simulink model "Ellipse"  (R2023a)
settings: Solver=FixedStepAuto  StartTime=0.0  StopTime=20  FixedStep=0.005  RelTol=1e-3
values from neighbouring files (symbols this model uses):
  step_height = 0.06    [InitialisationScript.m]    (also in simulation_setup.m)
  step_length = 0.04    [InitialisationScript.m]    (also in simulation_setup.m)
libraries: simulink_extras x2
settings Model: Creator=basti  LastModifiedBy=basti
settings SolverCC: EnableFixedStepZeroCrossing=on

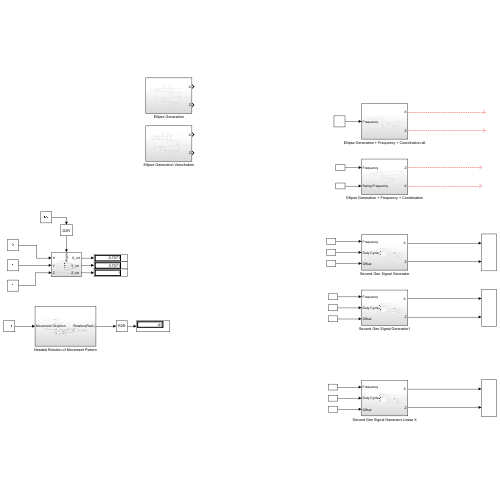
[thumbnail: Simulink's stored preview of the top-level diagram]
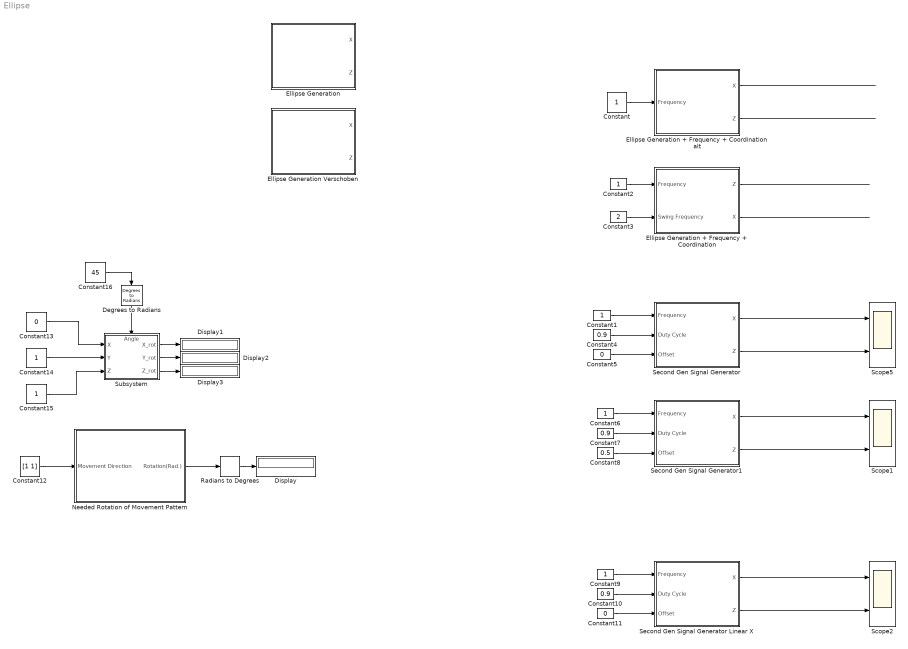
== system Ellipse ==
  Constant{,1..2,6,9,14..15} (7 alike) : Constant
  Constant10 : Constant  Value=0.9
  Constant11 : Constant  Value=0
  Constant12 : Constant  Value=[1 1]
  Constant13 : Constant  Value=0
  Constant16 : Constant  Value=45
  Constant3 : Constant  Value=2
  Constant4 : Constant  Value=0.9
  Constant5 : Constant  Value=0
  Constant7 : Constant  Value=0.9
  Constant8 : Constant  Value=0.5
  Degrees to Radians : simulink_extras/Transformations/Degrees to Radians
  Display{,1..3} (4 alike) : Display
  Ellipse Generation : Subsystem
  Ellipse Generation + Frequency + Coordination : Subsystem
  Ellipse Generation + Frequency + Coordination alt : Subsystem
  Ellipse Generation Verschoben : Subsystem
  Needed Rotation of Movement Pattern : Subsystem
  Radians to Degrees : simulink_extras/Transformations/Radians to Degrees
  Scope1 : Scope  NumInputPorts=2
  Scope2 : Scope  NumInputPorts=2
  Scope5 : Scope  NumInputPorts=2
  Second Gen Signal Generator : Subsystem
  Second Gen Signal Generator Linear X : Subsystem
  Second Gen Signal Generator1 : Subsystem
  Subsystem : Subsystem
      settings: PortSchema="{\"entries\":[{\"content\":{\"sides\":[{\"content\":{\"connectorIds\":[\"In1\",\"In2\",\"In3\"]},\"type\":\"ConnectorPlacement.EquallySpacedRectSide\",\"uuid\":\"84b9b2e7-3aec-4c44-82b0-943baf46ecad\"},{\"content\":{\"connectorIds\":[\"Out1\",\"Out2\",\"Out3\"],\"side\":\"RIGHT\"},\"type\":\"ConnectorPlacement.EquallySpacedRectSide\",\"uuid\":\"b6460351-c898-40bb-b6f7-4663874c85b4\"},{\"content\":{\"connectorIds\":[\"In4\"],\"side\":\"TOP\"},\"type\":\"ConnectorPlacement.EquallySpacedRectSide\",\"uuid\":\"52dfc046-6500-4cf8-9639-535088e7a0e1\"}]},\"type\":\"ConnectorPlacement.EquallySpacedConnector\",\"uuid\":\"f9a3b501-bdbb-45c4-9129-59c2d41cd802\"}],\"packageUris\":[\"http://schema.mathworks.com/mf0/Connector/R2020b\"],\"version\":\"1.0\"}"
  wires:
  Ellipse Generation + Frequency + Coordination alt/1(X) -> ?
  Ellipse Generation + Frequency + Coordination alt/2(Z) -> ?
  Constant/1 -> Ellipse Generation + Frequency + Coordination alt/1(Frequency)
  Constant3/1 -> Ellipse Generation + Frequency + Coordination/2(Swing Frequency)
  Constant2/1 -> Ellipse Generation + Frequency + Coordination/1(Frequency)
  Ellipse Generation + Frequency + Coordination/1(Z) -> ?
  Ellipse Generation + Frequency + Coordination/2(X) -> ?
  Constant1/1 -> Second Gen Signal Generator/1(Frequency)
  Constant4/1 -> Second Gen Signal Generator/2(Duty Cycle)
  Constant5/1 -> Second Gen Signal Generator/3(Offset)
  Second Gen Signal Generator/1("X ") -> Scope5/1
  Second Gen Signal Generator/2(Z) -> Scope5/2
  Constant6/1 -> Second Gen Signal Generator1/1(Frequency)
  Constant8/1 -> Second Gen Signal Generator1/3(Offset)
  Constant7/1 -> Second Gen Signal Generator1/2(Duty Cycle)
  Second Gen Signal Generator1/1("X ") -> Scope1/1
  Second Gen Signal Generator1/2(Z) -> Scope1/2
  Constant11/1 -> Second Gen Signal Generator Linear X/3(Offset)
  Constant10/1 -> Second Gen Signal Generator Linear X/2(Duty Cycle)
  Constant9/1 -> Second Gen Signal Generator Linear X/1(Frequency)
  Second Gen Signal Generator Linear X/2(Z) -> Scope2/2
  Second Gen Signal Generator Linear X/1("X ") -> Scope2/1
  Needed Rotation of Movement Pattern/1(Rotation(Rad.)) -> Radians to Degrees/1
  Radians to Degrees/1 -> Display/1
  Constant12/1 -> Needed Rotation of Movement Pattern/1(Movement Direction)
  Constant13/1 -> Subsystem/1("X ")
  Constant14/1 -> Subsystem/2(Y)
  Constant15/1 -> Subsystem/3(Z)
  Subsystem/1(X_rot) -> Display1/1
  Subsystem/2("Y_rot ") -> Display2/1
  Subsystem/3("Z_rot ") -> Display3/1
  Constant16/1 -> Degrees to Radians/1
  Degrees to Radians/1 -> Subsystem/4(Angle)

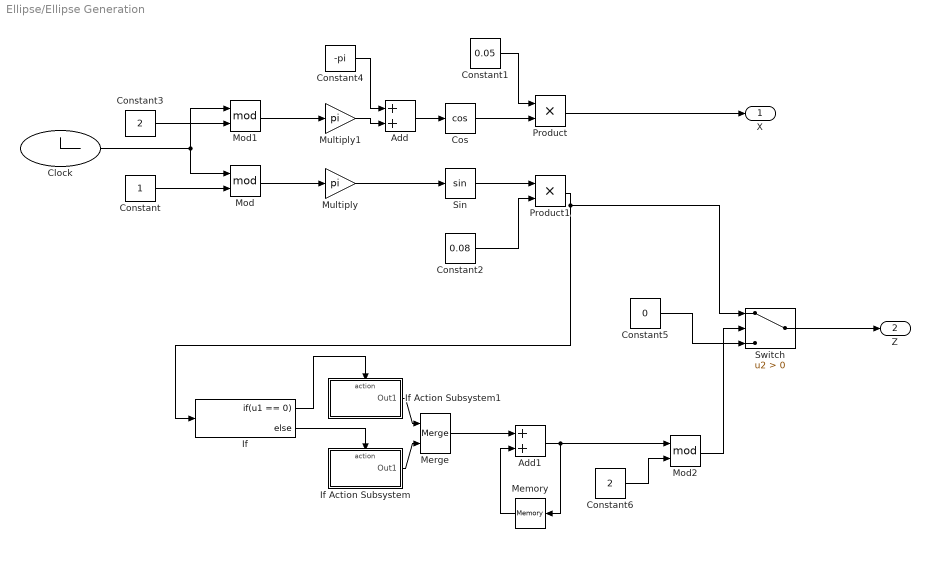
== system Ellipse/Ellipse Generation ==
  Add : Sum
  Add1 : Sum
  Clock : Clock
  Constant : Constant
  Constant1 : Constant  Value=0.05
  Constant2 : Constant  Value=0.08
  Constant3 : Constant  Value=2
  Constant4 : Constant  Value=-pi
  Constant5 : Constant  Value=0
  Constant6 : Constant  Value=2
  Cos : Trigonometry  Operator=cos
  If : If  IfExpression=u1 == 0
  If Action Subsystem : Subsystem  TreatAsAtomicUnit=on
  If Action Subsystem1 : Subsystem  TreatAsAtomicUnit=on
  Memory : Memory
  Merge : Merge
  Mod : Math  Operator=mod
  Mod1 : Math  Operator=mod
  Mod2 : Math  Operator=mod
  Multiply : Gain  Gain=pi
  Multiply1 : Gain  Gain=pi
  Product : Product
  Product1 : Product
  Sin : Trigonometry
  Switch : Switch  Criteria=u2 > Threshold  SaturateOnIntegerOverflow=off  InputSameDT=off
  X : Outport
  Z : Outport  Port=2
  wires:
  Clock/1 -> Mod1/1, Mod/1
  Constant/1 -> Mod/2
  Mod/1 -> Multiply/1
  Multiply/1 -> Sin/1
  Sin/1 -> Product1/1
  Cos/1 -> Product/2
  Constant1/1 -> Product/1
  Constant2/1 -> Product1/2
  Product1/1 -> Switch/1, If/1
  Product/1 -> X/1
  Mod1/1 -> Multiply1/1
  Constant3/1 -> Mod1/2
  Add/1 -> Cos/1
  Multiply1/1 -> Add/2
  Constant4/1 -> Add/1
  Add1/1 -> Mod2/1, Memory/1
  Memory/1 -> Add1/2
  If/2 -> If Action Subsystem/Action
  If/1 -> If Action Subsystem1/Action
  If Action Subsystem/1(Out1) -> Merge/2
  If Action Subsystem1/1(Out1) -> Merge/1
  Merge/1 -> Add1/1
  Switch/1 -> Z/1
  Constant5/1 -> Switch/3
  Constant6/1 -> Mod2/2
  Mod2/1 -> Switch/2

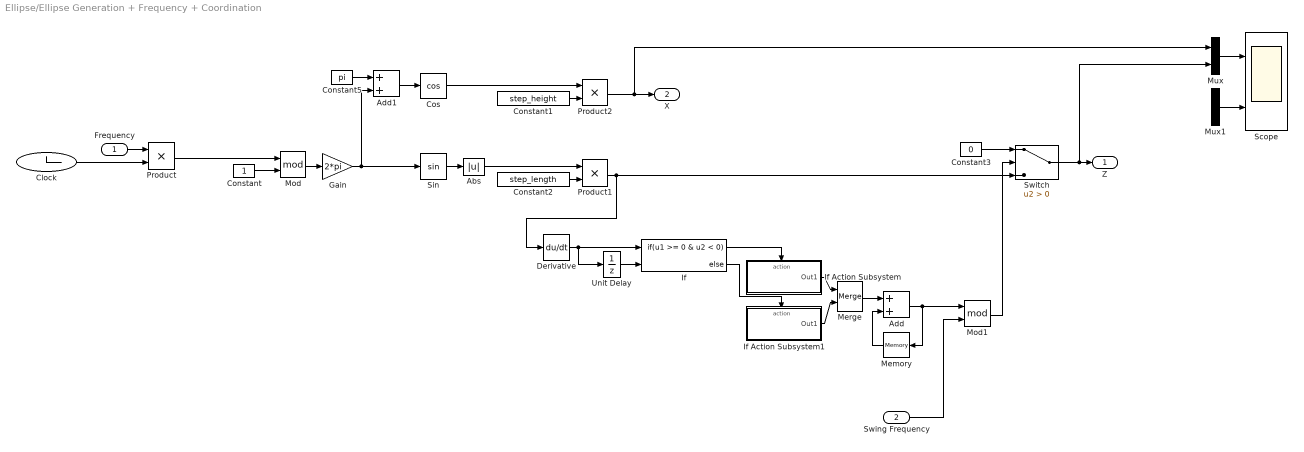
== system Ellipse/Ellipse Generation + Frequency + Coordination ==
  Frequency : Inport
  Swing Frequency : Inport  Port=2
  Abs : Abs  SaturateOnIntegerOverflow=off
  Add : Sum
  Add1 : Sum
  Clock : Clock
  Constant : Constant
  Constant1 : Constant  Value=step_height
  Constant2 : Constant  Value=step_length
  Constant3 : Constant  Value=0
  Constant5 : Constant  Value=pi
  Cos : Trigonometry  Operator=cos
  Derivative : Derivative
  Gain : Gain  Gain=2*pi
  If : If  NumInputs=2  IfExpression=u1 >= 0 & u2 < 0
  If Action Subsystem : Subsystem  TreatAsAtomicUnit=on
  If Action Subsystem1 : Subsystem  TreatAsAtomicUnit=on
  Memory : Memory
  Merge : Merge
  Mod : Math  Operator=mod
  Mod1 : Math  Operator=mod
  Mux : Mux  Inputs=2
  Mux1 : Mux  Inputs=2
  Product : Product
  Product1 : Product
  Product2 : Product
  Scope : Scope  NumInputPorts=2
  Sin : Trigonometry
  Switch : Switch  Criteria=u2 > Threshold  SaturateOnIntegerOverflow=off  InputSameDT=off
  Unit Delay : UnitDelay  SampleTime=-1  HasFrameUpgradeWarning=on
  Z : Outport
  X : Outport  Port=2
  wires:
  Clock/1 -> Product/2
  Frequency/1 -> Product/1
  Product/1 -> Mod/1
  Constant/1 -> Mod/2
  Mod/1 -> Gain/1
  Sin/1 -> Abs/1
  Constant2/1 -> Product1/2
  Cos/1 -> Product2/1
  Constant1/1 -> Product2/2
  Product1/1 -> Switch/3, Derivative/1
  Constant3/1 -> Switch/1
  Abs/1 -> Product1/1
  Derivative/1 -> Unit Delay/1, If/1
  Unit Delay/1 -> If/2
  If/2 -> If Action Subsystem1/Action
  If/1 -> If Action Subsystem/Action
  If Action Subsystem/1(Out1) -> Merge/1
  If Action Subsystem1/1(Out1) -> Merge/2
  Switch/1 -> Mux/2, Z/1
  Product2/1 -> Mux/1, X/1
  Merge/1 -> Add/1
  Memory/1 -> Add/2
  Add/1 -> Mod1/1, Memory/1
  Swing Frequency/1 -> Mod1/2
  Mod1/1 -> Switch/2
  Mux/1 -> Scope/1
  Mux1/1 -> Scope/2
  Add1/1 -> Cos/1
  Constant5/1 -> Add1/1
  Gain/1 -> Add1/2, Sin/1

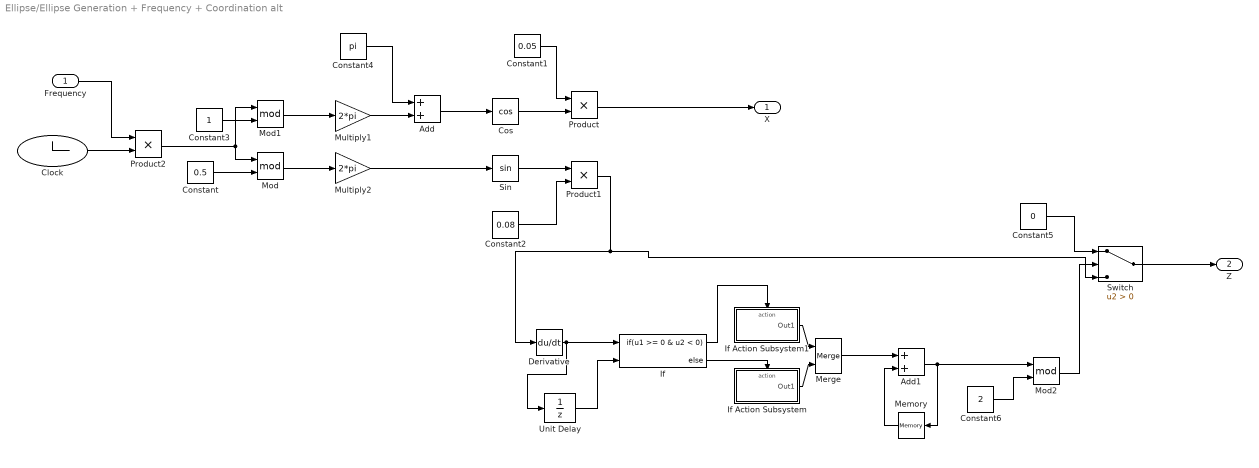
== system Ellipse/Ellipse Generation + Frequency + Coordination alt ==
  Frequency : Inport
  Add : Sum
  Add1 : Sum
  Clock : Clock
  Constant : Constant  Value=0.5
  Constant1 : Constant  Value=0.05
  Constant2 : Constant  Value=0.08
  Constant3 : Constant
  Constant4 : Constant  Value=pi
  Constant5 : Constant  Value=0
  Constant6 : Constant  Value=2
  Cos : Trigonometry  Operator=cos
  Derivative : Derivative
  If : If  NumInputs=2  IfExpression=u1 >= 0 & u2 < 0
  If Action Subsystem : Subsystem  TreatAsAtomicUnit=on
  If Action Subsystem1 : Subsystem  TreatAsAtomicUnit=on
  Memory : Memory
  Merge : Merge
  Mod : Math  Operator=mod
  Mod1 : Math  Operator=mod
  Mod2 : Math  Operator=mod
  Multiply1 : Gain  Gain=2*pi
  Multiply2 : Gain  Gain=2*pi
  Product : Product
  Product1 : Product
  Product2 : Product
  Sin : Trigonometry
  Switch : Switch  Criteria=u2 > Threshold  SaturateOnIntegerOverflow=off  InputSameDT=off
  Unit Delay : UnitDelay  SampleTime=-1  HasFrameUpgradeWarning=on
  X : Outport
  Z : Outport  Port=2
  wires:
  Constant/1 -> Mod/2
  Mod/1 -> Multiply2/1
  Sin/1 -> Product1/1
  Cos/1 -> Product/2
  Constant1/1 -> Product/1
  Constant2/1 -> Product1/2
  Product1/1 -> Derivative/1, Switch/3
  Product/1 -> X/1
  Mod1/1 -> Multiply1/1
  Constant3/1 -> Mod1/2
  Add1/1 -> Mod2/1, Memory/1
  Memory/1 -> Add1/2
  If/2 -> If Action Subsystem/Action
  If/1 -> If Action Subsystem1/Action
  If Action Subsystem/1(Out1) -> Merge/2
  If Action Subsystem1/1(Out1) -> Merge/1
  Switch/1 -> Z/1
  Constant5/1 -> Switch/1
  Constant6/1 -> Mod2/2
  Multiply1/1 -> Add/2
  Clock/1 -> Product2/2
  Derivative/1 -> Unit Delay/1, If/1
  Unit Delay/1 -> If/2
  Mod2/1 -> Switch/2
  Merge/1 -> Add1/1
  Constant4/1 -> Add/1
  Add/1 -> Cos/1
  Multiply2/1 -> Sin/1
  Product2/1 -> Mod/1, Mod1/1
  Frequency/1 -> Product2/1

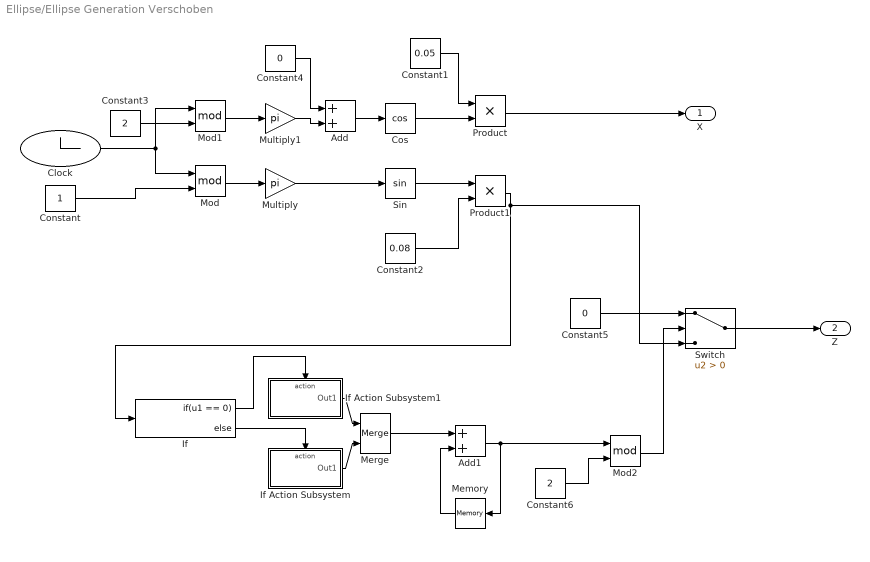
== system Ellipse/Ellipse Generation Verschoben ==
  Add : Sum
  Add1 : Sum
  Clock : Clock
  Constant : Constant
  Constant1 : Constant  Value=0.05
  Constant2 : Constant  Value=0.08
  Constant3 : Constant  Value=2
  Constant4 : Constant  Value=0
  Constant5 : Constant  Value=0
  Constant6 : Constant  Value=2
  Cos : Trigonometry  Operator=cos
  If : If  IfExpression=u1 == 0
  If Action Subsystem : Subsystem  TreatAsAtomicUnit=on
  If Action Subsystem1 : Subsystem  TreatAsAtomicUnit=on
  Memory : Memory
  Merge : Merge
  Mod : Math  Operator=mod
  Mod1 : Math  Operator=mod
  Mod2 : Math  Operator=mod
  Multiply : Gain  Gain=pi
  Multiply1 : Gain  Gain=pi
  Product : Product
  Product1 : Product
  Sin : Trigonometry
  Switch : Switch  Criteria=u2 > Threshold  SaturateOnIntegerOverflow=off  InputSameDT=off
  X : Outport
  Z : Outport  Port=2
  wires:
  Clock/1 -> Mod1/1, Mod/1
  Constant/1 -> Mod/2
  Mod/1 -> Multiply/1
  Multiply/1 -> Sin/1
  Sin/1 -> Product1/1
  Cos/1 -> Product/2
  Constant1/1 -> Product/1
  Constant2/1 -> Product1/2
  Product1/1 -> Switch/3, If/1
  Product/1 -> X/1
  Mod1/1 -> Multiply1/1
  Constant3/1 -> Mod1/2
  Add/1 -> Cos/1
  Multiply1/1 -> Add/2
  Constant4/1 -> Add/1
  Add1/1 -> Mod2/1, Memory/1
  Memory/1 -> Add1/2
  If/2 -> If Action Subsystem/Action
  If/1 -> If Action Subsystem1/Action
  If Action Subsystem/1(Out1) -> Merge/2
  If Action Subsystem1/1(Out1) -> Merge/1
  Merge/1 -> Add1/1
  Switch/1 -> Z/1
  Constant5/1 -> Switch/1
  Constant6/1 -> Mod2/2
  Mod2/1 -> Switch/2

== system Ellipse/Needed Rotation of Movement Pattern ==
  Movement Direction : Inport
  Atan2 : Trigonometry  Operator=atan2
  Constant12 : Constant  Commented=on  Value=[0 1]
  Gain : Gain  Gain=-1
  Product : Product
  Selector : Selector  Commented=on  IndexMode=Zero-based  InputPortWidth=2  IndexOptions=Starting index (dialog)  Indices=0  OutputSizes=1
  Selector1 : Selector  Commented=on  IndexMode=Zero-based  InputPortWidth=2  IndexOptions=Starting index (dialog)  Indices=1  OutputSizes=1
  Selector2 : Selector  IndexMode=Zero-based  InputPortWidth=2  IndexOptions=Starting index (dialog)  Indices=0  OutputSizes=1  RuntimeRangeChecks=on
  Selector3 : Selector  IndexMode=Zero-based  InputPortWidth=2  IndexOptions=Starting index (dialog)  Indices=1  OutputSizes=1
  Rotation(Rad.) : Outport
  wires:
  Product/1 -> Atan2/2
  Movement Direction/1 -> Selector3/1, Selector2/1
  Atan2/1 -> Rotation(Rad.)/1
  Constant12/1 -> Selector1/1, Selector/1
  Selector2/1 -> Gain/1, Product/1
  Gain/1 -> Atan2/1
  Selector3/1 -> Product/2

== system Ellipse/Second Gen Signal Generator ==
  note: (1/Hz) *duty_cycle = duty_cycle/Hz = swing_time
      |
      | 1/swing_time = 1 / (duty_cycle/Hz) = Hz/duty_cycle = Hz_for_swing
      | ----------------------------------------------------------------------------------------------------
      | (1/Hz)*(1-duty_cycle) = (1-duty_cycle)/Hz = stance_time
      |
      | 1/stance_time = 1 / ((1-duty_cycle)/Hz) = Hz / (1-duty_cycle) = Hz_for_stance
  Frequency : Inport
  Duty Cycle : Inport  Port=2
  Offset : Inport  Port=3
  Constant2 : Constant
  Divide : Product  Inputs=*/
  Divide1 : Product  Inputs=*/
  Gain : Gain  Gain=0.5
  Gain1 : Gain  Gain=0.5
  Stance Phase : Subsystem  TreatAsAtomicUnit=on
  Subsystem : Subsystem
  Subtract : Sum  Inputs=+-
  Swing Phase : Subsystem  TreatAsAtomicUnit=on
  Switch : Switch  Criteria=u2 > Threshold  SaturateOnIntegerOverflow=off  InputSameDT=off
  Switch1 : Switch  Criteria=u2 > Threshold  SaturateOnIntegerOverflow=off  InputSameDT=off
  "X " : Outport
  Z : Outport  Port=2
  wires:
  Swing Phase/1(X) -> Switch/1
  Swing Phase/2("Z ") -> Switch1/1
  Stance Phase/2("Z ") -> Switch1/3
  Stance Phase/1(X) -> Switch/3
  Divide1/1 -> Gain1/1
  Divide/1 -> Gain/1
  Duty Cycle/1 -> Subtract/2, Divide/2, Subsystem/2(Duty Cycle)
  Offset/1 -> Subsystem/3(Offset)
  Frequency/1 -> Divide1/1, Divide/1, Subsystem/1(Frequency)
  Subsystem/1(Swing Activation) -> Switch1/2, Switch/2, Swing Phase/Reset
  Subsystem/2(Stance Activation) -> Stance Phase/Reset
  Subtract/1 -> Divide1/2
  Constant2/1 -> Subtract/1
  Gain/1 -> Swing Phase/1(Frequency)
  Gain1/1 -> Stance Phase/1(Frequency)
  Switch1/1 -> Z/1
  Switch/1 -> "X "/1

== system Ellipse/Second Gen Signal Generator Linear X ==
  note: (1/Hz) *duty_cycle = duty_cycle/Hz = swing_time
      |
      | 1/swing_time = 1 / (duty_cycle/Hz) = Hz/duty_cycle = Hz_for_swing
      | ----------------------------------------------------------------------------------------------------
      | (1/Hz)*(1-duty_cycle) = (1-duty_cycle)/Hz = stance_time
      |
      | 1/stance_time = 1 / ((1-duty_cycle)/Hz) = Hz / (1-duty_cycle) = Hz_for_stance
  Frequency : Inport
  Duty Cycle : Inport  Port=2
  Offset : Inport  Port=3
  Constant2 : Constant
  Divide : Product  Inputs=*/
  Divide1 : Product  Inputs=*/
  Gain : Gain  Gain=0.5
  Gain1 : Gain  Gain=0.5
  Stance Phase : Subsystem  TreatAsAtomicUnit=on
  Subsystem : Subsystem
  Subtract : Sum  Inputs=+-
  Swing Phase : Subsystem  TreatAsAtomicUnit=on
  Switch : Switch  Criteria=u2 > Threshold  SaturateOnIntegerOverflow=off  InputSameDT=off
  Switch1 : Switch  Criteria=u2 > Threshold  SaturateOnIntegerOverflow=off  InputSameDT=off
  "X " : Outport
  Z : Outport  Port=2
  wires:
  Swing Phase/1(X) -> Switch/1
  Swing Phase/2("Z ") -> Switch1/1
  Stance Phase/2("Z ") -> Switch1/3
  Stance Phase/1(X) -> Switch/3
  Divide1/1 -> Gain1/1
  Divide/1 -> Gain/1
  Duty Cycle/1 -> Subtract/2, Divide/2, Subsystem/2(Duty Cycle)
  Offset/1 -> Subsystem/3(Offset)
  Frequency/1 -> Divide1/1, Divide/1, Subsystem/1(Frequency)
  Subsystem/1(Swing Activation) -> Switch1/2, Switch/2, Swing Phase/Reset
  Subsystem/2(Stance Activation) -> Stance Phase/Reset
  Subtract/1 -> Divide1/2
  Constant2/1 -> Subtract/1
  Gain/1 -> Swing Phase/1(Frequency)
  Gain1/1 -> Stance Phase/1(Frequency)
  Switch1/1 -> Z/1
  Switch/1 -> "X "/1

== system Ellipse/Second Gen Signal Generator1 ==
  note: (1/Hz) *duty_cycle = duty_cycle/Hz = swing_time
      |
      | 1/swing_time = 1 / (duty_cycle/Hz) = Hz/duty_cycle = Hz_for_swing
      | ----------------------------------------------------------------------------------------------------
      | (1/Hz)*(1-duty_cycle) = (1-duty_cycle)/Hz = stance_time
      |
      | 1/stance_time = 1 / ((1-duty_cycle)/Hz) = Hz / (1-duty_cycle) = Hz_for_stance
  Frequency : Inport
  Duty Cycle : Inport  Port=2
  Offset : Inport  Port=3
  Constant2 : Constant
  Divide : Product  Inputs=*/
  Divide1 : Product  Inputs=*/
  Gain : Gain  Gain=0.5
  Gain1 : Gain  Gain=0.5
  Stance Phase : Subsystem  TreatAsAtomicUnit=on
  Subsystem : Subsystem
  Subtract : Sum  Inputs=+-
  Swing Phase : Subsystem  TreatAsAtomicUnit=on
  Switch : Switch  Criteria=u2 > Threshold  SaturateOnIntegerOverflow=off  InputSameDT=off
  Switch1 : Switch  Criteria=u2 > Threshold  SaturateOnIntegerOverflow=off  InputSameDT=off
  "X " : Outport
  Z : Outport  Port=2
  wires:
  Swing Phase/1(X) -> Switch/1
  Swing Phase/2("Z ") -> Switch1/1
  Stance Phase/2("Z ") -> Switch1/3
  Stance Phase/1(X) -> Switch/3
  Divide1/1 -> Gain1/1
  Divide/1 -> Gain/1
  Duty Cycle/1 -> Subtract/2, Divide/2, Subsystem/2(Duty Cycle)
  Offset/1 -> Subsystem/3(Offset)
  Frequency/1 -> Divide1/1, Divide/1, Subsystem/1(Frequency)
  Subsystem/1(Swing Activation) -> Switch1/2, Switch/2, Swing Phase/Reset
  Subsystem/2(Stance Activation) -> Stance Phase/Reset
  Subtract/1 -> Divide1/2
  Constant2/1 -> Subtract/1
  Gain/1 -> Swing Phase/1(Frequency)
  Gain1/1 -> Stance Phase/1(Frequency)
  Switch1/1 -> Z/1
  Switch/1 -> "X "/1

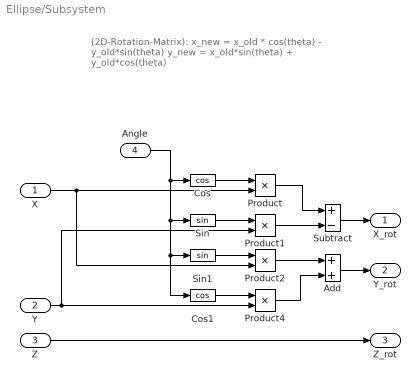
== system Ellipse/Subsystem ==
  note: (2D-Rotation-Matrix):
      | x_new = x_old * cos(theta) - y_old*sin(theta)
      | y_new = x_old*sin(theta) + y_old*cos(theta)
  "X " : Inport
  Y : Inport  Port=2
  Z : Inport  Port=3
  Angle : Inport  Port=4
  Add : Sum
  Cos : Trigonometry  Operator=cos
  Cos1 : Trigonometry  Operator=cos
  Product{,1..2,4} (4 alike) : Product
  Sin : Trigonometry
  Sin1 : Trigonometry
  Subtract : Sum  Inputs=+-
  X_rot : Outport
  "Y_rot " : Outport  Port=2
  "Z_rot " : Outport  Port=3
  wires:
  Z/1 -> "Z_rot "/1
  Subtract/1 -> X_rot/1
  Add/1 -> "Y_rot "/1
  Product/1 -> Subtract/1
  Product1/1 -> Subtract/2
  Product2/1 -> Add/1
  Product4/1 -> Add/2
  Cos/1 -> Product/1
  "X "/1 -> Product2/2, Product/2
  Angle/1 -> Cos1/1, Sin1/1, Sin/1, Cos/1
  Y/1 -> Product1/2, Product4/2
  Sin/1 -> Product1/1
  Sin1/1 -> Product2/1
  Cos1/1 -> Product4/1

== system Ellipse/Ellipse Generation/If Action Subsystem ==
  Action Port : ActionPort  ActionPortLabel=else
  Constant : Constant  Value=0
  Out1 : Outport
  wires:
  Constant/1 -> Out1/1

== system Ellipse/Ellipse Generation/If Action Subsystem1 ==
  Action Port : ActionPort  ActionPortLabel=if(u1 == 0)
  Constant : Constant
  Out1 : Outport
  wires:
  Constant/1 -> Out1/1

== system Ellipse/Ellipse Generation + Frequency + Coordination/If Action Subsystem ==
  Action Port : ActionPort  ActionPortLabel=if(u1 >= 0 & u2 < 0)
  Constant : Constant
  Out1 : Outport
  wires:
  Constant/1 -> Out1/1

== system Ellipse/Ellipse Generation + Frequency + Coordination/If Action Subsystem1 ==
  Action Port : ActionPort  ActionPortLabel=else
  Constant : Constant  Value=0
  Out1 : Outport
  wires:
  Constant/1 -> Out1/1

== system Ellipse/Ellipse Generation + Frequency + Coordination alt/If Action Subsystem ==
  Action Port : ActionPort  ActionPortLabel=else
  Constant : Constant  Value=0
  Out1 : Outport
  wires:
  Constant/1 -> Out1/1

== system Ellipse/Ellipse Generation + Frequency + Coordination alt/If Action Subsystem1 ==
  Action Port : ActionPort  ActionPortLabel=if(u1 >= 0 & u2 < 0)
  Constant : Constant
  Out1 : Outport
  wires:
  Constant/1 -> Out1/1

== system Ellipse/Ellipse Generation Verschoben/If Action Subsystem ==
  Action Port : ActionPort  ActionPortLabel=else
  Constant : Constant  Value=0
  Out1 : Outport
  wires:
  Constant/1 -> Out1/1

== system Ellipse/Ellipse Generation Verschoben/If Action Subsystem1 ==
  Action Port : ActionPort  ActionPortLabel=if(u1 == 0)
  Constant : Constant
  Out1 : Outport
  wires:
  Constant/1 -> Out1/1

== system Ellipse/Second Gen Signal Generator/Stance Phase ==
  Frequency : Inport
  Reset : ResetPort  DisableCoverage=on
  Add : Sum
  Constant : Constant
  Constant1 : Constant  Value=step_length
  Constant2 : Constant  Value=0
  Constant3 : Constant  Value=0.5*pi
  Constant4 : Constant  Value=-step_length
  Derivative : Derivative
  Gain : Gain  Gain=2*pi
  Integrator : Integrator
  Product : Product
  Product1 : Product
  Sin : Trigonometry
  Switch : Switch  Criteria=u2 > Threshold  SaturateOnIntegerOverflow=off  InputSameDT=off
  X : Outport
  "Z " : Outport  Port=2
  wires:
  Integrator/1 -> Gain/1
  Constant/1 -> Integrator/1
  Sin/1 -> Product/2
  Constant1/1 -> Product/1
  Constant2/1 -> "Z "/1
  Frequency/1 -> Product1/1
  Gain/1 -> Product1/2
  Add/1 -> Sin/1
  Product1/1 -> Add/2
  Constant3/1 -> Add/1
  Product/1 -> Derivative/1, Switch/3
  Switch/1 -> X/1
  Derivative/1 -> Switch/2
  Constant4/1 -> Switch/1

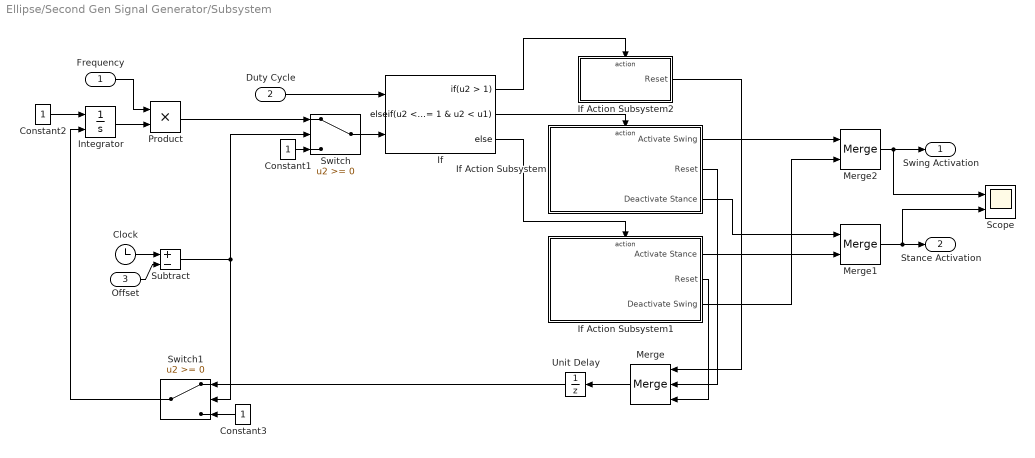
== system Ellipse/Second Gen Signal Generator/Subsystem ==
  Frequency : Inport
  Duty Cycle : Inport  Port=2
  Offset : Inport  Port=3
  Clock : Clock
  Constant1 : Constant
  Constant2 : Constant
  Constant3 : Constant
  If : If  NumInputs=2  IfExpression=u2 > 1  ElseIfExpressions=u2 <= 1 & u2 < u1
  If Action Subsystem : Subsystem  TreatAsAtomicUnit=on
  If Action Subsystem1 : Subsystem  TreatAsAtomicUnit=on
  If Action Subsystem2 : Subsystem  TreatAsAtomicUnit=on
  Integrator : Integrator  ExternalReset=level
  Merge : Merge  Inputs=3
  Merge1 : Merge
  Merge2 : Merge
  Product : Product
  Scope : Scope  NumInputPorts=2
  Subtract : Sum  Inputs=+-
  Switch : Switch  SaturateOnIntegerOverflow=off  InputSameDT=off
  Switch1 : Switch  SaturateOnIntegerOverflow=off  InputSameDT=off
  Unit Delay : UnitDelay  SampleTime=-1  HasFrameUpgradeWarning=on
  Swing Activation : Outport
  Stance Activation : Outport  Port=2
  wires:
  If Action Subsystem/3(Deactivate Stance) -> Merge1/1
  If/2 -> If Action Subsystem/Action
  Duty Cycle/1 -> If/1
  If/1 -> If Action Subsystem2/Action
  If Action Subsystem1/1(Activate Stance) -> Merge1/2
  If Action Subsystem/2(Reset) -> Merge/2
  Merge/1 -> Unit Delay/1
  If Action Subsystem1/3(Deactivate Swing) -> Merge2/2
  If Action Subsystem2/1(Reset) -> Merge/1
  If Action Subsystem/1(Activate Swing) -> Merge2/1
  If Action Subsystem1/2(Reset) -> Merge/3
  If/3 -> If Action Subsystem1/Action
  Merge2/1 -> Scope/1, Swing Activation/1
  Merge1/1 -> Scope/2, Stance Activation/1
  Switch/1 -> If/2
  Constant1/1 -> Switch/3
  Subtract/1 -> Switch1/2, Switch/2
  Offset/1 -> Subtract/2
  Clock/1 -> Subtract/1
  Integrator/1 -> Product/2
  Product/1 -> Switch/1
  Frequency/1 -> Product/1
  Constant2/1 -> Integrator/1
  Unit Delay/1 -> Switch1/1
  Constant3/1 -> Switch1/3
  Switch1/1 -> Integrator/2

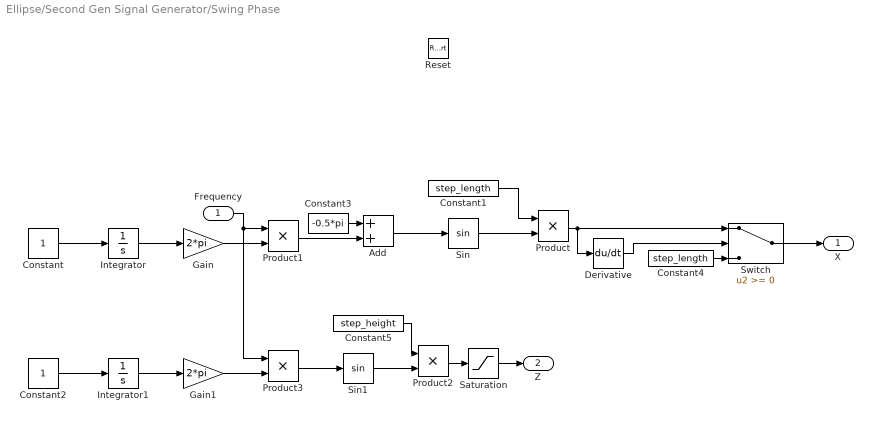
== system Ellipse/Second Gen Signal Generator/Swing Phase ==
  Frequency : Inport
  Reset : ResetPort  DisableCoverage=on
  Add : Sum
  Constant : Constant
  Constant1 : Constant  Value=step_length
  Constant2 : Constant
  Constant3 : Constant  Value=-0.5*pi
  Constant4 : Constant  Value=step_length
  Constant5 : Constant  Value=step_height
  Derivative : Derivative
  Gain : Gain  Gain=2*pi
  Gain1 : Gain  Gain=2*pi
  Integrator : Integrator
  Integrator1 : Integrator
  Product{,1..3} (4 alike) : Product
  Saturation : Saturate  UpperLimit=step_height  LowerLimit=0
  Sin : Trigonometry
  Sin1 : Trigonometry
  Switch : Switch  SaturateOnIntegerOverflow=off  InputSameDT=off
  X : Outport
  "Z " : Outport  Port=2
  wires:
  Integrator/1 -> Gain/1
  Constant/1 -> Integrator/1
  Sin/1 -> Product/2
  Constant1/1 -> Product/1
  Product2/1 -> Saturation/1
  Gain/1 -> Product1/2
  Add/1 -> Sin/1
  Product1/1 -> Add/2
  Constant3/1 -> Add/1
  Product/1 -> Switch/1, Derivative/1
  Constant4/1 -> Switch/3
  Switch/1 -> X/1
  Derivative/1 -> Switch/2
  Product3/1 -> Sin1/1
  Sin1/1 -> Product2/2
  Constant5/1 -> Product2/1
  Constant2/1 -> Integrator1/1
  Gain1/1 -> Product3/2
  Integrator1/1 -> Gain1/1
  Frequency/1 -> Product3/1, Product1/1
  Saturation/1 -> "Z "/1

== system Ellipse/Second Gen Signal Generator Linear X/Stance Phase ==
  Frequency : Inport
  Reset : ResetPort  DisableCoverage=on
  Add : Sum
  Constant1 : Constant  Value=step_length
  Constant2 : Constant  Value=0
  Constant5 : Constant  Value=step_length
  Constant6 : Constant
  Gain1 : Gain  Gain=-4
  Integrator1 : Integrator
  Product2 : Product
  Product3 : Product
  Saturation : Saturate  UpperLimit=step_length  LowerLimit=-step_length
  X : Outport
  "Z " : Outport  Port=2
  wires:
  Constant2/1 -> "Z "/1
  Constant5/1 -> Add/1
  Constant6/1 -> Integrator1/1
  Add/1 -> Saturation/1
  Product3/1 -> Add/2
  Integrator1/1 -> Product3/2
  Frequency/1 -> Product2/2
  Gain1/1 -> Product2/1
  Product2/1 -> Product3/1
  Saturation/1 -> X/1
  Constant1/1 -> Gain1/1

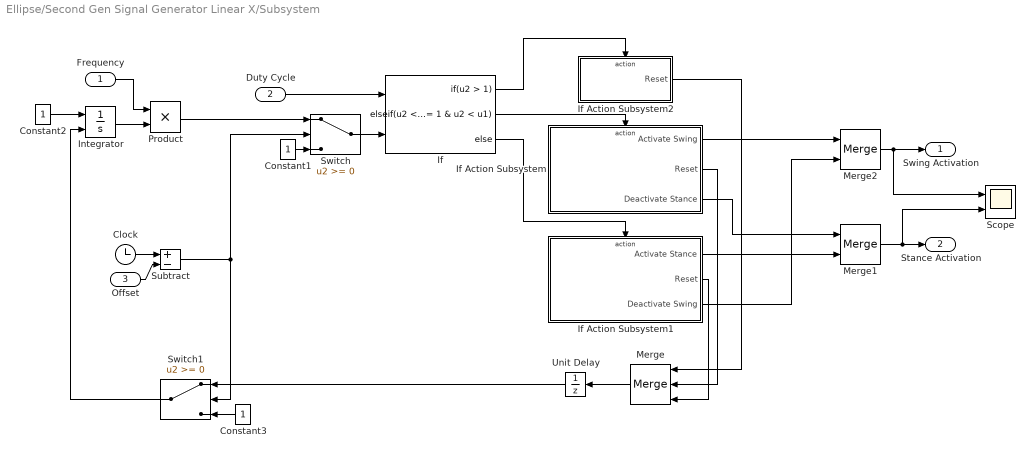
== system Ellipse/Second Gen Signal Generator Linear X/Subsystem ==
  Frequency : Inport
  Duty Cycle : Inport  Port=2
  Offset : Inport  Port=3
  Clock : Clock
  Constant1 : Constant
  Constant2 : Constant
  Constant3 : Constant
  If : If  NumInputs=2  IfExpression=u2 > 1  ElseIfExpressions=u2 <= 1 & u2 < u1
  If Action Subsystem : Subsystem  TreatAsAtomicUnit=on
  If Action Subsystem1 : Subsystem  TreatAsAtomicUnit=on
  If Action Subsystem2 : Subsystem  TreatAsAtomicUnit=on
  Integrator : Integrator  ExternalReset=level
  Merge : Merge  Inputs=3
  Merge1 : Merge
  Merge2 : Merge
  Product : Product
  Scope : Scope  NumInputPorts=2
  Subtract : Sum  Inputs=+-
  Switch : Switch  SaturateOnIntegerOverflow=off  InputSameDT=off
  Switch1 : Switch  SaturateOnIntegerOverflow=off  InputSameDT=off
  Unit Delay : UnitDelay  SampleTime=-1  HasFrameUpgradeWarning=on
  Swing Activation : Outport
  Stance Activation : Outport  Port=2
  wires:
  If Action Subsystem/3(Deactivate Stance) -> Merge1/1
  If/2 -> If Action Subsystem/Action
  Duty Cycle/1 -> If/1
  If/1 -> If Action Subsystem2/Action
  If Action Subsystem1/1(Activate Stance) -> Merge1/2
  If Action Subsystem/2(Reset) -> Merge/2
  Merge/1 -> Unit Delay/1
  If Action Subsystem1/3(Deactivate Swing) -> Merge2/2
  If Action Subsystem2/1(Reset) -> Merge/1
  If Action Subsystem/1(Activate Swing) -> Merge2/1
  If Action Subsystem1/2(Reset) -> Merge/3
  If/3 -> If Action Subsystem1/Action
  Merge2/1 -> Scope/1, Swing Activation/1
  Merge1/1 -> Scope/2, Stance Activation/1
  Switch/1 -> If/2
  Constant1/1 -> Switch/3
  Subtract/1 -> Switch1/2, Switch/2
  Offset/1 -> Subtract/2
  Clock/1 -> Subtract/1
  Integrator/1 -> Product/2
  Product/1 -> Switch/1
  Frequency/1 -> Product/1
  Constant2/1 -> Integrator/1
  Unit Delay/1 -> Switch1/1
  Constant3/1 -> Switch1/3
  Switch1/1 -> Integrator/2

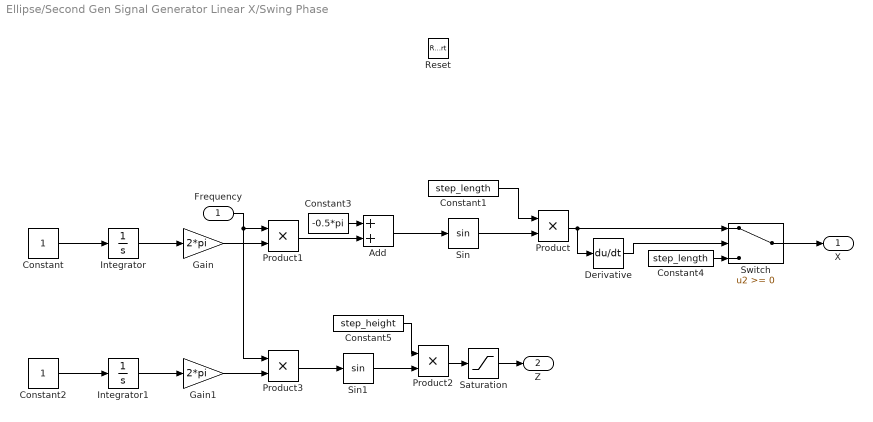
== system Ellipse/Second Gen Signal Generator Linear X/Swing Phase ==
  Frequency : Inport
  Reset : ResetPort  DisableCoverage=on
  Add : Sum
  Constant : Constant
  Constant1 : Constant  Value=step_length
  Constant2 : Constant
  Constant3 : Constant  Value=-0.5*pi
  Constant4 : Constant  Value=step_length
  Constant5 : Constant  Value=step_height
  Derivative : Derivative
  Gain : Gain  Gain=2*pi
  Gain1 : Gain  Gain=2*pi
  Integrator : Integrator
  Integrator1 : Integrator
  Product{,1..3} (4 alike) : Product
  Saturation : Saturate  UpperLimit=step_height  LowerLimit=0
  Sin : Trigonometry
  Sin1 : Trigonometry
  Switch : Switch  SaturateOnIntegerOverflow=off  InputSameDT=off
  X : Outport
  "Z " : Outport  Port=2
  wires:
  Integrator/1 -> Gain/1
  Constant/1 -> Integrator/1
  Sin/1 -> Product/2
  Constant1/1 -> Product/1
  Product2/1 -> Saturation/1
  Gain/1 -> Product1/2
  Add/1 -> Sin/1
  Product1/1 -> Add/2
  Constant3/1 -> Add/1
  Product/1 -> Switch/1, Derivative/1
  Constant4/1 -> Switch/3
  Switch/1 -> X/1
  Derivative/1 -> Switch/2
  Product3/1 -> Sin1/1
  Sin1/1 -> Product2/2
  Constant5/1 -> Product2/1
  Constant2/1 -> Integrator1/1
  Gain1/1 -> Product3/2
  Integrator1/1 -> Gain1/1
  Frequency/1 -> Product3/1, Product1/1
  Saturation/1 -> "Z "/1

== system Ellipse/Second Gen Signal Generator1/Stance Phase ==
  Frequency : Inport
  Reset : ResetPort  DisableCoverage=on
  Add : Sum
  Constant : Constant
  Constant1 : Constant  Value=step_length
  Constant2 : Constant  Value=0
  Constant3 : Constant  Value=0.5*pi
  Constant4 : Constant  Value=-step_length
  Derivative : Derivative
  Gain : Gain  Gain=2*pi
  Integrator : Integrator
  Product : Product
  Product1 : Product
  Sin : Trigonometry
  Switch : Switch  Criteria=u2 > Threshold  SaturateOnIntegerOverflow=off  InputSameDT=off
  X : Outport
  "Z " : Outport  Port=2
  wires:
  Integrator/1 -> Gain/1
  Constant/1 -> Integrator/1
  Sin/1 -> Product/2
  Constant1/1 -> Product/1
  Constant2/1 -> "Z "/1
  Frequency/1 -> Product1/1
  Gain/1 -> Product1/2
  Add/1 -> Sin/1
  Product1/1 -> Add/2
  Constant3/1 -> Add/1
  Product/1 -> Derivative/1, Switch/3
  Switch/1 -> X/1
  Derivative/1 -> Switch/2
  Constant4/1 -> Switch/1

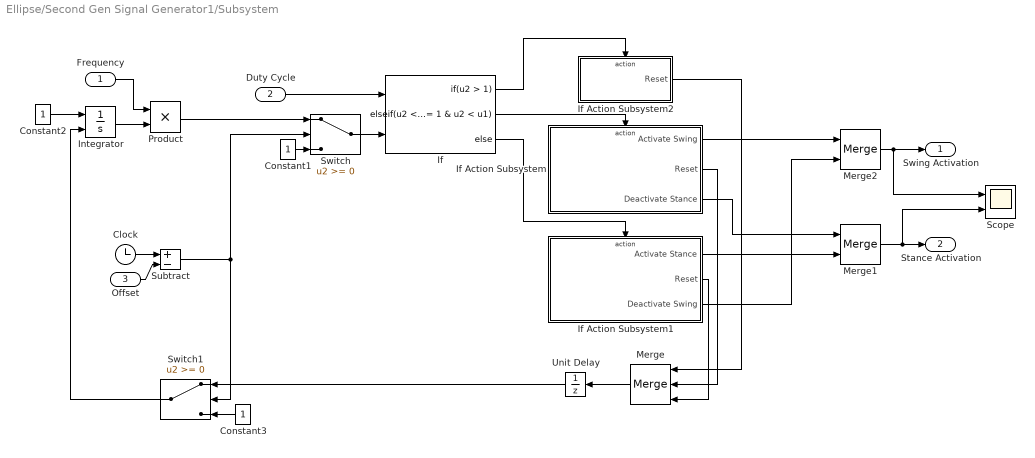
== system Ellipse/Second Gen Signal Generator1/Subsystem ==
  Frequency : Inport
  Duty Cycle : Inport  Port=2
  Offset : Inport  Port=3
  Clock : Clock
  Constant1 : Constant
  Constant2 : Constant
  Constant3 : Constant
  If : If  NumInputs=2  IfExpression=u2 > 1  ElseIfExpressions=u2 <= 1 & u2 < u1
  If Action Subsystem : Subsystem  TreatAsAtomicUnit=on
  If Action Subsystem1 : Subsystem  TreatAsAtomicUnit=on
  If Action Subsystem2 : Subsystem  TreatAsAtomicUnit=on
  Integrator : Integrator  ExternalReset=level
  Merge : Merge  Inputs=3
  Merge1 : Merge
  Merge2 : Merge
  Product : Product
  Scope : Scope  NumInputPorts=2
  Subtract : Sum  Inputs=+-
  Switch : Switch  SaturateOnIntegerOverflow=off  InputSameDT=off
  Switch1 : Switch  SaturateOnIntegerOverflow=off  InputSameDT=off
  Unit Delay : UnitDelay  SampleTime=-1  HasFrameUpgradeWarning=on
  Swing Activation : Outport
  Stance Activation : Outport  Port=2
  wires:
  If Action Subsystem/3(Deactivate Stance) -> Merge1/1
  If/2 -> If Action Subsystem/Action
  Duty Cycle/1 -> If/1
  If/1 -> If Action Subsystem2/Action
  If Action Subsystem1/1(Activate Stance) -> Merge1/2
  If Action Subsystem/2(Reset) -> Merge/2
  Merge/1 -> Unit Delay/1
  If Action Subsystem1/3(Deactivate Swing) -> Merge2/2
  If Action Subsystem2/1(Reset) -> Merge/1
  If Action Subsystem/1(Activate Swing) -> Merge2/1
  If Action Subsystem1/2(Reset) -> Merge/3
  If/3 -> If Action Subsystem1/Action
  Merge2/1 -> Scope/1, Swing Activation/1
  Merge1/1 -> Scope/2, Stance Activation/1
  Switch/1 -> If/2
  Constant1/1 -> Switch/3
  Subtract/1 -> Switch1/2, Switch/2
  Offset/1 -> Subtract/2
  Clock/1 -> Subtract/1
  Integrator/1 -> Product/2
  Product/1 -> Switch/1
  Frequency/1 -> Product/1
  Constant2/1 -> Integrator/1
  Unit Delay/1 -> Switch1/1
  Constant3/1 -> Switch1/3
  Switch1/1 -> Integrator/2

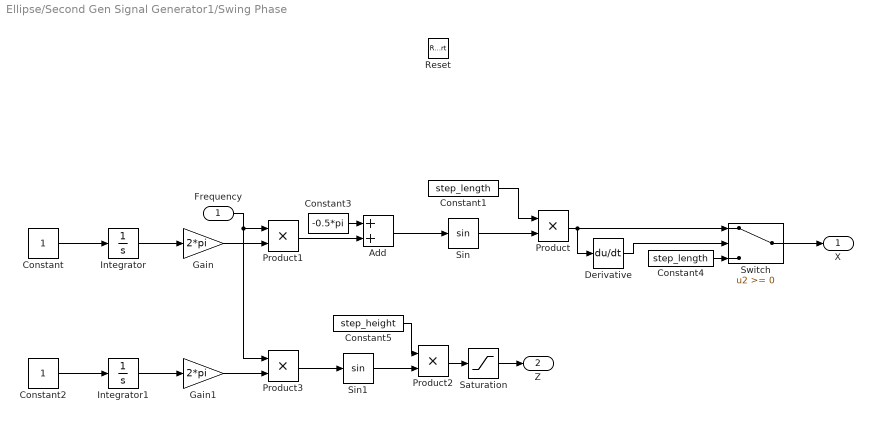
== system Ellipse/Second Gen Signal Generator1/Swing Phase ==
  Frequency : Inport
  Reset : ResetPort  DisableCoverage=on
  Add : Sum
  Constant : Constant
  Constant1 : Constant  Value=step_length
  Constant2 : Constant
  Constant3 : Constant  Value=-0.5*pi
  Constant4 : Constant  Value=step_length
  Constant5 : Constant  Value=step_height
  Derivative : Derivative
  Gain : Gain  Gain=2*pi
  Gain1 : Gain  Gain=2*pi
  Integrator : Integrator
  Integrator1 : Integrator
  Product{,1..3} (4 alike) : Product
  Saturation : Saturate  UpperLimit=step_height  LowerLimit=0
  Sin : Trigonometry
  Sin1 : Trigonometry
  Switch : Switch  SaturateOnIntegerOverflow=off  InputSameDT=off
  X : Outport
  "Z " : Outport  Port=2
  wires:
  Integrator/1 -> Gain/1
  Constant/1 -> Integrator/1
  Sin/1 -> Product/2
  Constant1/1 -> Product/1
  Product2/1 -> Saturation/1
  Gain/1 -> Product1/2
  Add/1 -> Sin/1
  Product1/1 -> Add/2
  Constant3/1 -> Add/1
  Product/1 -> Switch/1, Derivative/1
  Constant4/1 -> Switch/3
  Switch/1 -> X/1
  Derivative/1 -> Switch/2
  Product3/1 -> Sin1/1
  Sin1/1 -> Product2/2
  Constant5/1 -> Product2/1
  Constant2/1 -> Integrator1/1
  Gain1/1 -> Product3/2
  Integrator1/1 -> Gain1/1
  Frequency/1 -> Product3/1, Product1/1
  Saturation/1 -> "Z "/1

== system Ellipse/Second Gen Signal Generator/Subsystem/If Action Subsystem ==
  Action Port : ActionPort  ActionPortLabel=elseif(u2 <= 1 & u2 < u1)
  Constant : Constant
  Constant1 : Constant  Value=0
  Constant2 : Constant  Value=0
  Activate Swing : Outport
  Reset : Outport  Port=2
  Deactivate Stance : Outport  Port=3
  wires:
  Constant/1 -> Activate Swing/1
  Constant1/1 -> Reset/1
  Constant2/1 -> Deactivate Stance/1

== system Ellipse/Second Gen Signal Generator/Subsystem/If Action Subsystem1 ==
  Action Port : ActionPort  ActionPortLabel=else
  Constant : Constant
  Constant1 : Constant  Value=0
  Constant2 : Constant  Value=0
  Activate Stance : Outport
  Reset : Outport  Port=2
  Deactivate Swing : Outport  Port=3
  wires:
  Constant/1 -> Activate Stance/1
  Constant1/1 -> Reset/1
  Constant2/1 -> Deactivate Swing/1

== system Ellipse/Second Gen Signal Generator/Subsystem/If Action Subsystem2 ==
  Action Port : ActionPort  ActionPortLabel=if(u2 > 1)
  Constant1 : Constant
  Reset : Outport
  wires:
  Constant1/1 -> Reset/1

== system Ellipse/Second Gen Signal Generator Linear X/Subsystem/If Action Subsystem ==
  Action Port : ActionPort  ActionPortLabel=elseif(u2 <= 1 & u2 < u1)
  Constant : Constant
  Constant1 : Constant  Value=0
  Constant2 : Constant  Value=0
  Activate Swing : Outport
  Reset : Outport  Port=2
  Deactivate Stance : Outport  Port=3
  wires:
  Constant/1 -> Activate Swing/1
  Constant1/1 -> Reset/1
  Constant2/1 -> Deactivate Stance/1

== system Ellipse/Second Gen Signal Generator Linear X/Subsystem/If Action Subsystem1 ==
  Action Port : ActionPort  ActionPortLabel=else
  Constant : Constant
  Constant1 : Constant  Value=0
  Constant2 : Constant  Value=0
  Activate Stance : Outport
  Reset : Outport  Port=2
  Deactivate Swing : Outport  Port=3
  wires:
  Constant/1 -> Activate Stance/1
  Constant1/1 -> Reset/1
  Constant2/1 -> Deactivate Swing/1

== system Ellipse/Second Gen Signal Generator Linear X/Subsystem/If Action Subsystem2 ==
  Action Port : ActionPort  ActionPortLabel=if(u2 > 1)
  Constant1 : Constant
  Reset : Outport
  wires:
  Constant1/1 -> Reset/1

== system Ellipse/Second Gen Signal Generator1/Subsystem/If Action Subsystem ==
  Action Port : ActionPort  ActionPortLabel=elseif(u2 <= 1 & u2 < u1)
  Constant : Constant
  Constant1 : Constant  Value=0
  Constant2 : Constant  Value=0
  Activate Swing : Outport
  Reset : Outport  Port=2
  Deactivate Stance : Outport  Port=3
  wires:
  Constant/1 -> Activate Swing/1
  Constant1/1 -> Reset/1
  Constant2/1 -> Deactivate Stance/1

== system Ellipse/Second Gen Signal Generator1/Subsystem/If Action Subsystem1 ==
  Action Port : ActionPort  ActionPortLabel=else
  Constant : Constant
  Constant1 : Constant  Value=0
  Constant2 : Constant  Value=0
  Activate Stance : Outport
  Reset : Outport  Port=2
  Deactivate Swing : Outport  Port=3
  wires:
  Constant/1 -> Activate Stance/1
  Constant1/1 -> Reset/1
  Constant2/1 -> Deactivate Swing/1

== system Ellipse/Second Gen Signal Generator1/Subsystem/If Action Subsystem2 ==
  Action Port : ActionPort  ActionPortLabel=if(u2 > 1)
  Constant1 : Constant
  Reset : Outport
  wires:
  Constant1/1 -> Reset/1
